simulink model "Scheme5"  (R2023b)
settings: Solver=FixedStepAuto  StartTime=0.0  StopTime=10.0  FixedStep=0.001  RelTol=1e-3
libraries: commdigbbndpm3 x2, commchan3 x1, commsink2 x1, simulink_extras x1, dspfdesign x1
settings Model: Creator=User  LastModifiedBy=User

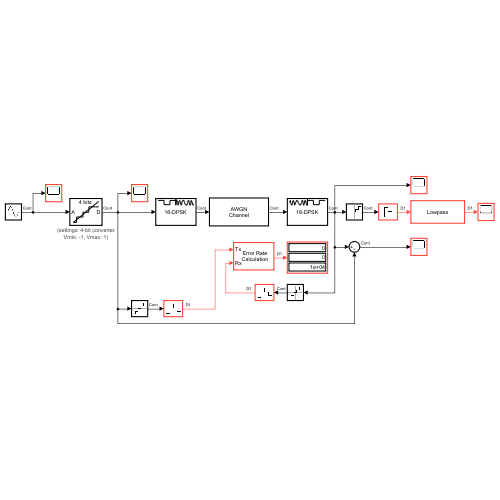
[thumbnail: Simulink's stored preview of the top-level diagram]
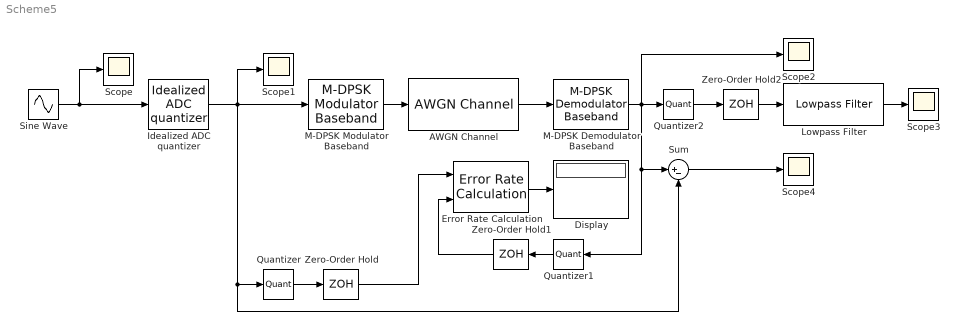
== system Scheme5 ==
  AWGN Channel : commchan3/AWGN Channel  LegacyMode=off  NoiseMethod="Signal to noise ratio  (SNR)"  noiseMode="Signal to noise ratio  (SNR)"  EbNo=10  EsNo=10  SNR=50  BitsPerSymbol=1  SignalPower=1  SamplesPerSymbol=1  SymbolPeriod=1  VarianceSource=Parameter  Variance=1  RandomStream=Global stream  Seed=67  SimulateUsing=Code generation
  Display : Display
  Error Rate Calculation : commsink2/Error Rate Calculation  N=0  st_delay=0  cp_mode=Entire frame  subframe=[]  PMode=Port  WsName=ErrorVec  RsMode2=off  stop=off  numErr=100  maxBits=1e6
  Idealized ADC quantizer : simulink_extras/Additional Discrete/Idealized ADC quantizer  NumberOfConverterBits=4  Vmin=-1  Vmax=1  OutputDataType=double  OutputNegativeValues=off
  Lowpass Filter : dspfdesign/Lowpass Filter  FilterType=FIR  DesignForMinimumOrder=on  FilterOrder=50  PassbandFrequency=8e3  StopbandFrequency=12e3  PassbandRipple=0.2  StopbandAttenuation=80  SampleRateMode=Specify on dialog  SampleRate=44100  SimulateUsing=Interpreted execution  roundingMode=Floor  coeffsDataTypeStr=fixdt(1,16)
  M-DPSK Demodulator Baseband : commdigbbndpm3/M-DPSK Demodulator Baseband  M=16  OutType=Integer  Dec=Gray  Ph=pi/16  outDtype1=Inherit via internal rule  outDtype2=Inherit via internal rule
  M-DPSK Modulator Baseband : commdigbbndpm3/M-DPSK Modulator Baseband  M=16  InType=Integer  Enc=Gray  Ph=pi/16  outDtype=double
  Quantizer : Quantizer
  Quantizer1 : Quantizer
  Quantizer2 : Quantizer
  Scope{,1..4} (5 alike) : Scope
  Sine Wave : Sin  Frequency=2  SampleTime=0
  Sum : Sum  Inputs=|+-
  Zero-Order Hold : ZeroOrderHold  SampleTime=-1
  Zero-Order Hold1 : ZeroOrderHold  SampleTime=-1
  Zero-Order Hold2 : ZeroOrderHold  SampleTime=-1
  wires:
  M-DPSK Modulator Baseband/1 -> AWGN Channel/1
  Idealized ADC quantizer/1 -> M-DPSK Modulator Baseband/1, Quantizer/1, Sum/2, Scope1/1
  M-DPSK Demodulator Baseband/1 -> Scope2/1, Quantizer1/1, Sum/1, Quantizer2/1
  Sum/1 -> Scope4/1
  Sine Wave/1 -> Scope/1, Idealized ADC quantizer/1
  Lowpass Filter/1 -> Scope3/1
  Error Rate Calculation/1 -> Display/1
  Quantizer/1 -> Zero-Order Hold/1
  Zero-Order Hold/1 -> Error Rate Calculation/1
  Quantizer1/1 -> Zero-Order Hold1/1
  Zero-Order Hold1/1 -> Error Rate Calculation/2
  Quantizer2/1 -> Zero-Order Hold2/1
  Zero-Order Hold2/1 -> Lowpass Filter/1
  AWGN Channel/1 -> M-DPSK Demodulator Baseband/1
